simulink model "sysgen_oversample2x_2samples_per_clock"  (R2016b)
settings: Solver=VariableStepAuto  StartTime=0.0  StopTime=samples_per_channel*number_channels  RelTol=1e-3
PreLoadFcn:
  | setup
values from neighbouring files (symbols this model uses):
  filts = reshape(filt,number_subband,taps_per_chan)    [setup.m]
undefined symbols (not defined in the file or in its folder): j
libraries: xbsIndex_r4 x186, dspsigops x4, dspxfrm3 x4, hdlsllib x2
(part 1 of 3)
settings Model: Creator=mdewart  LastModifiedBy=mdewart

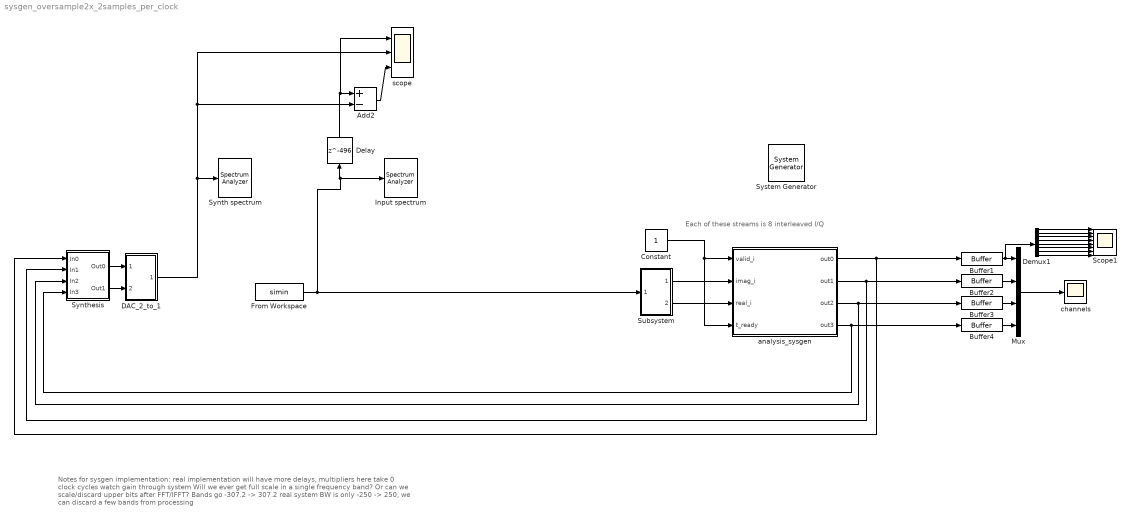
== system sysgen_oversample2x_2samples_per_clock ==
  note: Notes for sysgen implementation:
      |
      | real implementation will have more delays, multipliers here take 0 clock cycles
      |
      | watch gain through system
      |      Will we ever get full scale in a single frequency band?  Or can we scale/discard upper bits after FFT/IFFT?
      |
      | Bands go -307.2 -> 307.2  real system BW is only -250 -> 250, we can discard a few bands from processing
  note: Each of these streams is 8 interleaved I/Q
  " System Generator" : xbsIndex_r4/ System Generator  Tag=genX  xilinxfamily=kintexu  part=xcku040  speed=-2-e  package=ffva1156  synthesis_tool=Vivado  clock_wrapper=Clock Enables  directory=./netlist  proj_type=Vivado  Synth_file=Vivado Synthesis Defaults  Impl_file=Vivado Implementation Defaults  testbench=off  simulink_period=2  sysclk_period=10  dcm_input_clock_period=10  incr_netlist=off  trim_vbits=Everywhere in SubSystem  dbl_ovrd=According to Block Masks  core_generation=According to Block Masks  run_coregen=off  deprecated_control=off  eval_field=0  block_type=sysgen
  Add2 : Sum  Inputs=+-
  Buffer{1..4} (4 alike) : Buffer  N=8  TreatMby1Signals=One channel  OutputFrames=off
  Constant : Constant  SampleTime=2
  DAC_2_to_1 : Subsystem
  Delay : Delay  DelayLength=496  InitialCondition=0
  Demux1 : Demux  Outputs=8
  From Workspace : FromWorkspace  VariableName=simin  SampleTime=1  Interpolate=off  OutputAfterFinalValue=Cyclic repetition
  Input spectrum : SpectrumAnalyzer
  Mux : Mux
  Scope1 : Scope  NumInputPorts=8
  Subsystem : Subsystem
  Synth spectrum : SpectrumAnalyzer
  Synthesis : Subsystem
  analysis_sysgen : Subsystem
  channels : Scope
  scope : Scope  NumInputPorts=3
  wires:
  Mux/1 -> channels/1
  Buffer2/1 -> Mux/2
  Buffer3/1 -> Mux/3
  Buffer4/1 -> Mux/4
  Add2/1 -> scope/3
  DAC_2_to_1/1(Out1) -> Add2/2, scope/2, Synth spectrum/1
  Delay/1 -> Add2/1, scope/1
  Subsystem/1(imag) -> analysis_sysgen/2(imag_i)
  Subsystem/2(real) -> analysis_sysgen/3(real_i)
  Constant/1 -> analysis_sysgen/4(t_ready), analysis_sysgen/1(valid_i)
  Buffer1/1 -> Demux1/1, Mux/1
  From Workspace/1 -> Delay/1, Input spectrum/1, Subsystem/1(In1)
  Demux1/1 -> Scope1/1
  Demux1/2 -> Scope1/2
  Demux1/3 -> Scope1/3
  Demux1/4 -> Scope1/4
  Demux1/5 -> Scope1/5
  Demux1/6 -> Scope1/6
  Demux1/7 -> Scope1/7
  Demux1/8 -> Scope1/8
  analysis_sysgen/3(out2) -> Buffer3/1, Synthesis/3(In2)
  analysis_sysgen/4(out3) -> Synthesis/4(In3), Buffer4/1
  analysis_sysgen/2(out1) -> Buffer2/1, Synthesis/2(In1)
  analysis_sysgen/1(out0) -> Buffer1/1, Synthesis/1(In0)
  Synthesis/1(Out0) -> DAC_2_to_1/1(In1)
  Synthesis/2(Out1) -> DAC_2_to_1/2(In2)

== system sysgen_oversample2x_2samples_per_clock/DAC_2_to_1 ==
  In1 : Inport
  In2 : Inport  Port=2
  Add2 : Sum
  Delay7 : Delay  DelayLength=1  InitialCondition=0
  Upsample1 : dspsigops/Upsample  N=2  phase=0  RateOptions=Allow multirate processing  ic=0  mode=Unused parameter value
  Upsample2 : dspsigops/Upsample  N=2  phase=0  RateOptions=Allow multirate processing  ic=0  mode=Unused parameter value
  Out1 : Outport
  wires:
  In2/1 -> Upsample2/1
  Delay7/1 -> Add2/2
  In1/1 -> Upsample1/1
  Upsample1/1 -> Add2/1
  Add2/1 -> Out1/1
  Upsample2/1 -> Delay7/1

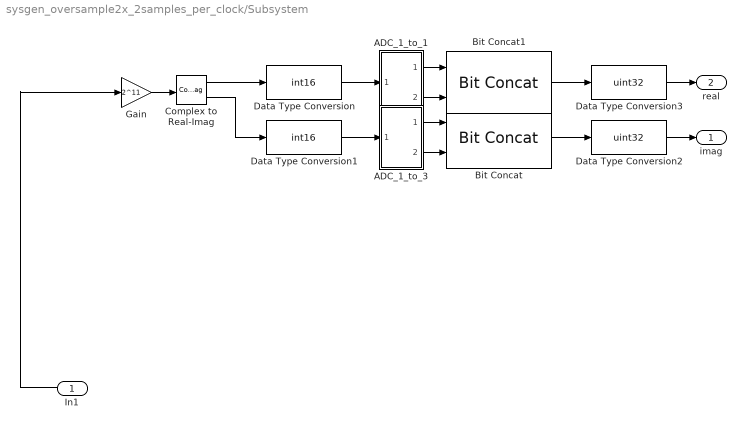
== system sysgen_oversample2x_2samples_per_clock/Subsystem ==
  In1 : Inport
  ADC_1_to_1 : Subsystem
  ADC_1_to_3 : Subsystem
  Bit Concat : hdlsllib/HDL Operations/Bit Concat  numInputs=2
  Bit Concat1 : hdlsllib/HDL Operations/Bit Concat  numInputs=2
  Complex to Real-Imag : ComplexToRealImag
  Data Type Conversion : DataTypeConversion  OutDataTypeStr=int16
  Data Type Conversion1 : DataTypeConversion  OutDataTypeStr=int16
  Data Type Conversion2 : DataTypeConversion  OutDataTypeStr=uint32  ConvertRealWorld=Stored Integer (SI)
  Data Type Conversion3 : DataTypeConversion  OutDataTypeStr=uint32  ConvertRealWorld=Stored Integer (SI)
  Gain : Gain  Gain=2^11
  imag : Outport
  real : Outport  Port=2
  wires:
  In1/1 -> Gain/1
  Data Type Conversion/1 -> ADC_1_to_1/1(In1)
  Complex to Real-Imag/1 -> Data Type Conversion/1
  ADC_1_to_3/2(Out2) -> Bit Concat/2
  Data Type Conversion1/1 -> ADC_1_to_3/1(In1)
  ADC_1_to_1/1(Out1) -> Bit Concat1/1
  Bit Concat/1 -> Data Type Conversion2/1
  ADC_1_to_3/1(Out1) -> Bit Concat/1
  ADC_1_to_1/2(Out2) -> Bit Concat1/2
  Complex to Real-Imag/2 -> Data Type Conversion1/1
  Gain/1 -> Complex to Real-Imag/1
  Bit Concat1/1 -> Data Type Conversion3/1
  Data Type Conversion2/1 -> imag/1
  Data Type Conversion3/1 -> real/1

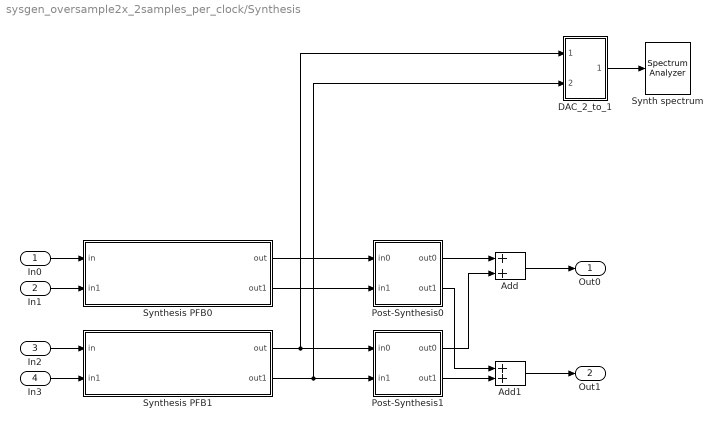
== system sysgen_oversample2x_2samples_per_clock/Synthesis ==
  In0 : Inport
  In1 : Inport  Port=2
  In2 : Inport  Port=3
  In3 : Inport  Port=4
  Add : Sum
  Add1 : Sum
  DAC_2_to_1 : Subsystem
  Post-Synthesis0 : Subsystem
  Post-Synthesis1 : Subsystem
  Synth spectrum : SpectrumAnalyzer
  Synthesis PFB0 : Subsystem
  Synthesis PFB1 : Subsystem
  Out0 : Outport
  Out1 : Outport  Port=2
  wires:
  Synthesis PFB0/2(out1) -> Post-Synthesis0/2(in1)
  Synthesis PFB0/1(out) -> Post-Synthesis0/1(in0)
  Post-Synthesis1/1(out0) -> Add/2
  Post-Synthesis0/2(out1) -> Add1/1
  Synthesis PFB1/2(out1) -> DAC_2_to_1/2(In2), Post-Synthesis1/2(in1)
  Post-Synthesis1/2(out1) -> Add1/2
  Synthesis PFB1/1(out) -> DAC_2_to_1/1(In1), Post-Synthesis1/1(in0)
  In2/1 -> Synthesis PFB1/1(in)
  In3/1 -> Synthesis PFB1/2(in1)
  In0/1 -> Synthesis PFB0/1(in)
  In1/1 -> Synthesis PFB0/2(in1)
  Post-Synthesis0/1(out0) -> Add/1
  Add1/1 -> Out1/1
  Add/1 -> Out0/1
  DAC_2_to_1/1(Out1) -> Synth spectrum/1

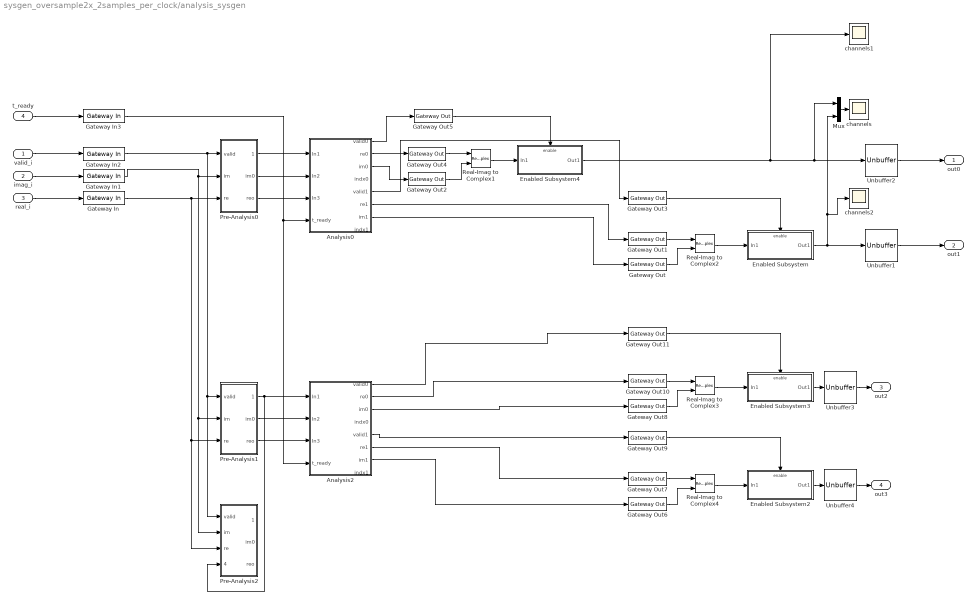
== system sysgen_oversample2x_2samples_per_clock/analysis_sysgen ==
  valid_i : Inport
  imag_i : Inport  Port=2
  real_i : Inport  Port=3
  t_ready : Inport  Port=4
  Analysis0 : Subsystem
  Analysis2 : Subsystem
  Enabled Subsystem : Subsystem  TreatAsAtomicUnit=on
  Enabled Subsystem2 : Subsystem  TreatAsAtomicUnit=on
  Enabled Subsystem3 : Subsystem  TreatAsAtomicUnit=on
  Enabled Subsystem4 : Subsystem  TreatAsAtomicUnit=on
  Gateway In : xbsIndex_r4/Gateway In  gui_display_data_type=Fixed-point  arith_type=Unsigned  n_bits=32  bin_pt=0  preci_type=Single  exp_width=8  frac_width=24  rows=1  columns=1  quantization="Round  (unbiased: +/- Inf)"  overflow=Saturate  period=2  UseAsADC=off  ADCChannel='1'  interface=None  automatic_assignment=on  address_offset=hex2dec('00')  intf_name=''  intf_description=''  default_value=0  timing_constraint=None  locs_specified=off  LOCs={}  io_standard={}  inherit_from_input=off  hdl_port=on  dbl_ovrd=off  block_type=gatewayin
  Gateway In1 : xbsIndex_r4/Gateway In  gui_display_data_type=Fixed-point  arith_type=Unsigned  n_bits=32  bin_pt=0  preci_type=Single  exp_width=8  frac_width=24  rows=1  columns=1  quantization="Round  (unbiased: +/- Inf)"  overflow=Saturate  period=2  UseAsADC=off  ADCChannel='1'  interface=None  automatic_assignment=on  address_offset=hex2dec('00')  intf_name=''  intf_description=''  default_value=0  timing_constraint=None  locs_specified=off  LOCs={}  io_standard={}  inherit_from_input=off  hdl_port=on  dbl_ovrd=off  block_type=gatewayin
  Gateway In2 : xbsIndex_r4/Gateway In  gui_display_data_type=Boolean  arith_type=Boolean  n_bits=1  bin_pt=0  preci_type=Single  exp_width=8  frac_width=24  rows=1  columns=1  quantization="Round  (unbiased: +/- Inf)"  overflow=Saturate  period=2  UseAsADC=off  ADCChannel='1'  interface=None  automatic_assignment=on  address_offset=hex2dec('00')  intf_name=''  intf_description=''  default_value=0  timing_constraint=None  locs_specified=off  LOCs={}  io_standard={}  inherit_from_input=off  hdl_port=on  dbl_ovrd=off  block_type=gatewayin
  Gateway In3 : xbsIndex_r4/Gateway In  gui_display_data_type=Boolean  arith_type=Boolean  n_bits=1  bin_pt=0  preci_type=Single  exp_width=8  frac_width=24  rows=1  columns=1  quantization="Round  (unbiased: +/- Inf)"  overflow=Saturate  period=2  UseAsADC=off  ADCChannel='1'  interface=None  automatic_assignment=on  address_offset=hex2dec('00')  intf_name=''  intf_description=''  default_value=0  timing_constraint=None  locs_specified=off  LOCs={}  io_standard={}  inherit_from_input=off  hdl_port=on  dbl_ovrd=off  block_type=gatewayin
  Gateway Out{,1..11} (12 alike) : xbsIndex_r4/Gateway Out  inherit_from_input=off  hdl_port=off  rows=1  columns=1  UseAsDAC=off  DACChannel='1'  interface=None  automatic_assignment=on  address_offset=hex2dec('00')  intf_name=''  intf_description=''  timing_constraint=None  locs_specified=off  LOCs={}  io_standard={}  block_type=gatewayout
  Mux : Mux  Inputs=2
  Pre-Analysis0 : Subsystem
  Pre-Analysis1 : Subsystem
  Pre-Analysis2 : Subsystem
  Real-Imag to Complex{1..4} (4 alike) : RealImagToComplex
  Unbuffer{1..4} (4 alike) : Unbuffer  SampleBasedProcessing=Same as frame based
  channels : Scope
  channels1 : Scope
  channels2 : Scope
  out0 : Outport
  out1 : Outport  Port=2
  out2 : Outport  Port=3
  out3 : Outport  Port=4
  wires:
  valid_i/1 -> Gateway In2/1
  t_ready/1 -> Gateway In3/1
  real_i/1 -> Gateway In/1
  imag_i/1 -> Gateway In1/1
  Enabled Subsystem/1(Out1) -> channels2/1, Mux/2, Unbuffer1/1
  Gateway Out1/1 -> Real-Imag to Complex2/1
  Gateway Out/1 -> Real-Imag to Complex2/2
  Real-Imag to Complex2/1 -> Enabled Subsystem/1(In1)
  Gateway Out3/1 -> Enabled Subsystem/Enable
  Gateway Out4/1 -> Real-Imag to Complex1/1
  Gateway Out2/1 -> Real-Imag to Complex1/2
  Analysis0/5(valid1) -> Gateway Out3/1
  Analysis0/6(re1) -> Gateway Out1/1
  Analysis0/7(im1) -> Gateway Out/1
  Gateway Out7/1 -> Real-Imag to Complex4/1
  Gateway Out6/1 -> Real-Imag to Complex4/2
  Real-Imag to Complex4/1 -> Enabled Subsystem2/1(In1)
  Gateway Out9/1 -> Enabled Subsystem2/Enable
  Gateway Out10/1 -> Real-Imag to Complex3/1
  Gateway Out8/1 -> Real-Imag to Complex3/2
  Gateway Out11/1 -> Enabled Subsystem3/Enable
  Real-Imag to Complex3/1 -> Enabled Subsystem3/1(In1)
  Analysis2/1(valid0) -> Gateway Out11/1
  Analysis2/2(re0) -> Gateway Out10/1
  Analysis2/5(valid1) -> Gateway Out9/1
  Gateway In2/1 -> Pre-Analysis1/1(valid), Pre-Analysis2/1(valid), Pre-Analysis0/1(valid)
  Gateway In1/1 -> Pre-Analysis1/2(im), Pre-Analysis2/2(im), Pre-Analysis0/2(im)
  Gateway In/1 -> Pre-Analysis2/3(re), Pre-Analysis1/3(re), Pre-Analysis0/3(re)
  Pre-Analysis0/3(reo) -> Analysis0/3(In3)
  Pre-Analysis0/2(im0) -> Analysis0/2(In2)
  Pre-Analysis0/1(valid0) -> Analysis0/1(In1)
  Gateway In3/1 -> Analysis2/4(t_ready), Analysis0/4(t_ready)
  Pre-Analysis1/3(reo) -> Analysis2/3(In3)
  Pre-Analysis1/2(im0) -> Analysis2/2(In2)
  Pre-Analysis1/1(valid0) -> Analysis2/1(In1), Pre-Analysis2/4(valid1)
  Real-Imag to Complex1/1 -> Enabled Subsystem4/1(In1)
  Gateway Out5/1 -> Enabled Subsystem4/Enable
  Unbuffer2/1 -> out0/1
  Unbuffer1/1 -> out1/1
  Enabled Subsystem3/1(Out1) -> Unbuffer3/1
  Unbuffer3/1 -> out2/1
  Enabled Subsystem2/1(Out1) -> Unbuffer4/1
  Unbuffer4/1 -> out3/1
  Analysis0/3(im0) -> Gateway Out2/1
  Analysis0/2(re0) -> Gateway Out4/1
  Analysis0/1(valid0) -> Gateway Out5/1
  Mux/1 -> channels/1
  Enabled Subsystem4/1(Out1) -> channels1/1, Mux/1, Unbuffer2/1
  Analysis2/3(im0) -> Gateway Out8/1
  Analysis2/6(re1) -> Gateway Out7/1
  Analysis2/7(im1) -> Gateway Out6/1

== system sysgen_oversample2x_2samples_per_clock/Subsystem/ADC_1_to_1 ==
  In1 : Inport
  Delay1 : Delay  DelayLength=1  InitialCondition=0
  Downsample : DownSample  RateOptions=Allow multirate processing
  Downsample1 : DownSample  RateOptions=Allow multirate processing
  Out1 : Outport
  Out2 : Outport  Port=2
  wires:
  Downsample/1 -> Out2/1
  In1/1 -> Downsample/1, Delay1/1
  Downsample1/1 -> Out1/1
  Delay1/1 -> Downsample1/1

== system sysgen_oversample2x_2samples_per_clock/Subsystem/ADC_1_to_3 ==
  In1 : Inport
  Delay1 : Delay  DelayLength=1  InitialCondition=0
  Downsample : DownSample  RateOptions=Allow multirate processing
  Downsample1 : DownSample  RateOptions=Allow multirate processing
  Out1 : Outport
  Out2 : Outport  Port=2
  wires:
  Delay1/1 -> Downsample1/1
  Downsample1/1 -> Out1/1
  In1/1 -> Delay1/1, Downsample/1
  Downsample/1 -> Out2/1

== system sysgen_oversample2x_2samples_per_clock/Synthesis/DAC_2_to_1 ==
  In1 : Inport
  In2 : Inport  Port=2
  Add2 : Sum
  Delay7 : Delay  DelayLength=1  InitialCondition=0
  Upsample1 : dspsigops/Upsample  N=2  phase=0  RateOptions=Allow multirate processing  ic=0  mode=Unused parameter value
  Upsample2 : dspsigops/Upsample  N=2  phase=0  RateOptions=Allow multirate processing  ic=0  mode=Unused parameter value
  Out1 : Outport
  wires:
  In2/1 -> Upsample2/1
  Delay7/1 -> Add2/2
  In1/1 -> Upsample1/1
  Upsample1/1 -> Add2/1
  Add2/1 -> Out1/1
  Upsample2/1 -> Delay7/1

== system sysgen_oversample2x_2samples_per_clock/Synthesis/Post-Synthesis0 ==
  note: Post-synthesis0 match timing to post-synthesis
  in0 : Inport
  in1 : Inport  Port=2
  out0 : Outport
  out1 : Outport  Port=2
  wires:
  in1/1 -> out1/1
  in0/1 -> out0/1

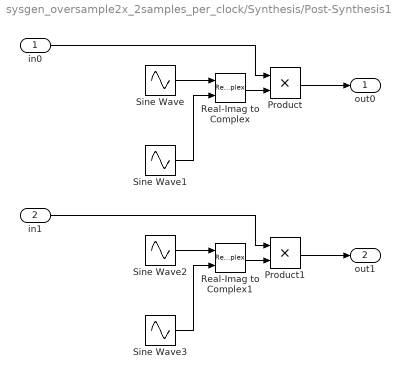
== system sysgen_oversample2x_2samples_per_clock/Synthesis/Post-Synthesis1 ==
  in0 : Inport
  in1 : Inport  Port=2
  Product : Product
  Product1 : Product
  Real-Imag to Complex : RealImagToComplex
  Real-Imag to Complex1 : RealImagToComplex
  Sine Wave : Sin  Frequency=2*pi/32  Phase=-pi/2  SampleTime=2
  Sine Wave1 : Sin  Amplitude=-1  Frequency=2*pi/32  SampleTime=2
  Sine Wave2 : Sin  Frequency=2*pi/32  Phase=-pi/2+pi/16  SampleTime=2
  Sine Wave3 : Sin  Amplitude=-1  Frequency=2*pi/32  Phase=0+pi/16  SampleTime=2
  out0 : Outport
  out1 : Outport  Port=2
  wires:
  in0/1 -> Product/1
  ? -> ?
  ? -> ?
  Sine Wave/1 -> Real-Imag to Complex/1
  Sine Wave1/1 -> Real-Imag to Complex/2
  in1/1 -> Product1/1
  Sine Wave2/1 -> Real-Imag to Complex1/1
  Sine Wave3/1 -> Real-Imag to Complex1/2
  Real-Imag to Complex1/1 -> Product1/2
  Real-Imag to Complex/1 -> Product/2
  Product1/1 -> out1/1
  Product/1 -> out0/1

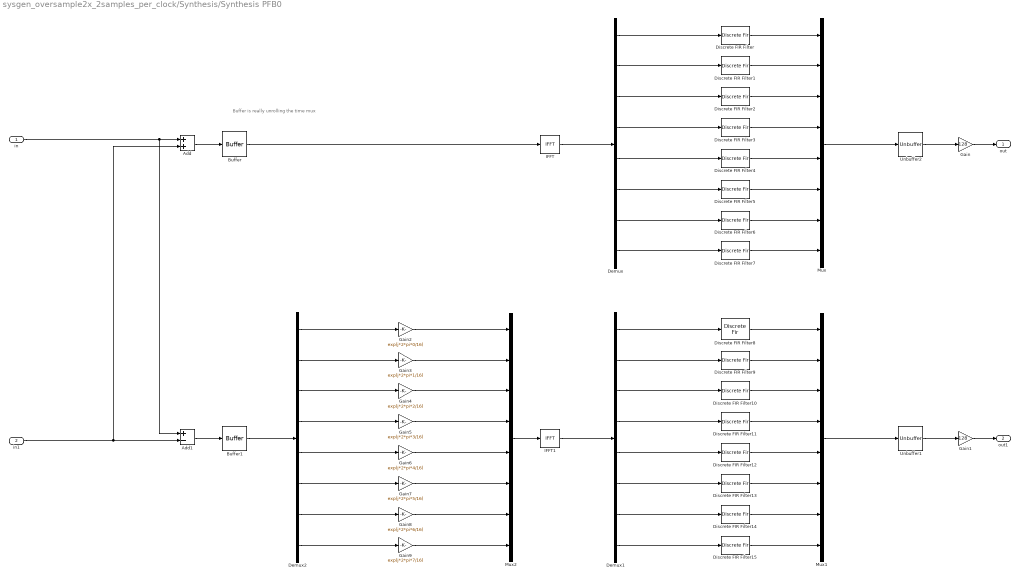
== system sysgen_oversample2x_2samples_per_clock/Synthesis/Synthesis PFB0 ==
  note: Buffer is really unrolling the time mux
  in : Inport
  in1 : Inport  Port=2
  Add : Sum
  Add1 : Sum  Inputs=+-
  Buffer : Buffer  N=8  TreatMby1Signals=One channel  OutputFrames=off
  Buffer1 : Buffer  N=8  TreatMby1Signals=One channel  OutputFrames=off
  Demux : Demux  Outputs=8
  Demux1 : Demux  Outputs=8
  Demux2 : Demux  Outputs=8
  Discrete FIR Filter : DiscreteFir  Coefficients=filts(1,:)
  Discrete FIR Filter1 : DiscreteFir  Coefficients=filts(3,:)
  Discrete FIR Filter10 : DiscreteFir  Coefficients=filts(6,:)
  Discrete FIR Filter11 : DiscreteFir  Coefficients=filts(8,:)
  Discrete FIR Filter12 : DiscreteFir  Coefficients=filts(10,:)
  Discrete FIR Filter13 : DiscreteFir  Coefficients=filts(12,:)
  Discrete FIR Filter14 : DiscreteFir  Coefficients=filts(14,:)
  Discrete FIR Filter15 : DiscreteFir  Coefficients=filts(16,:)
  Discrete FIR Filter2 : DiscreteFir  Coefficients=filts(5,:)
  Discrete FIR Filter3 : DiscreteFir  Coefficients=filts(7,:)
  Discrete FIR Filter4 : DiscreteFir  Coefficients=filts(9,:)
  Discrete FIR Filter5 : DiscreteFir  Coefficients=filts(11,:)
  Discrete FIR Filter6 : DiscreteFir  Coefficients=filts(13,:)
  Discrete FIR Filter7 : DiscreteFir  Coefficients=filts(15,:)
  Discrete FIR Filter8 : DiscreteFir  Coefficients=filts(2,:)
  Discrete FIR Filter9 : DiscreteFir  Coefficients=filts(4,:)
  Gain : Gain  Gain=128
  Gain1 : Gain  Gain=128
  Gain2 : Gain  Gain=exp(j*2*pi*0/16)
  Gain3 : Gain  Gain=exp(j*2*pi*1/16)
  Gain4 : Gain  Gain=exp(j*2*pi*2/16)
  Gain5 : Gain  Gain=exp(j*2*pi*3/16)
  Gain6 : Gain  Gain=exp(j*2*pi*4/16)
  Gain7 : Gain  Gain=exp(j*2*pi*5/16)
  Gain8 : Gain  Gain=exp(j*2*pi*6/16)
  Gain9 : Gain  Gain=exp(j*2*pi*7/16)
  IFFT : dspxfrm3/IFFT  FFTImplementation=Auto  CompMethod=Table lookup  TableOpt=NEW  TableOptActive=Speed  BitRevOrder=off  cs_in=off  Normalize=on  InheritFFTLength=on  FFTLength=64  WrapInput=on  mode=Complex  outSamplingMode=Sample based  roundingMode=Floor  overflowMode=off  firstCoeffDataTypeStr=Inherit: Same word length as input  firstCoeffLastDataTypeStr=Inherit: Same word length as input  outputMin=[]  outputMax=[]
  IFFT1 : dspxfrm3/IFFT  FFTImplementation=Auto  CompMethod=Table lookup  TableOpt=NEW  TableOptActive=Speed  BitRevOrder=off  cs_in=off  Normalize=on  InheritFFTLength=on  FFTLength=64  WrapInput=on  mode=Complex  outSamplingMode=Sample based  roundingMode=Floor  overflowMode=off  firstCoeffDataTypeStr=Inherit: Same word length as input  firstCoeffLastDataTypeStr=Inherit: Same word length as input  outputMin=[]  outputMax=[]
  Mux : Mux  Inputs=8
  Mux1 : Mux  Inputs=8
  Mux2 : Mux  Inputs=8
  Unbuffer1 : Unbuffer  SampleBasedProcessing=Same as frame based
  Unbuffer2 : Unbuffer  SampleBasedProcessing=Same as frame based
  out : Outport
  out1 : Outport  Port=2
  wires:
  Discrete FIR Filter7/1 -> Mux/8
  IFFT/1 -> Demux/1
  Demux/2 -> Discrete FIR Filter1/1
  Demux/7 -> Discrete FIR Filter6/1
  Demux/5 -> Discrete FIR Filter4/1
  Demux/8 -> Discrete FIR Filter7/1
  Demux/3 -> Discrete FIR Filter2/1
  Demux/1 -> Discrete FIR Filter/1
  Demux/6 -> Discrete FIR Filter5/1
  Discrete FIR Filter5/1 -> Mux/6
  Discrete FIR Filter/1 -> Mux/1
  Discrete FIR Filter4/1 -> Mux/5
  Discrete FIR Filter2/1 -> Mux/3
  Discrete FIR Filter1/1 -> Mux/2
  Discrete FIR Filter3/1 -> Mux/4
  Discrete FIR Filter6/1 -> Mux/7
  Demux/4 -> Discrete FIR Filter3/1
  Mux/1 -> Unbuffer2/1
  Unbuffer2/1 -> Gain/1
  Add/1 -> Buffer/1
  in/1 -> Add1/1, Add/1
  Discrete FIR Filter15/1 -> Mux1/8
  IFFT1/1 -> Demux1/1
  Demux1/2 -> Discrete FIR Filter9/1
  Demux1/7 -> Discrete FIR Filter14/1
  Demux1/5 -> Discrete FIR Filter12/1
  Demux1/8 -> Discrete FIR Filter15/1
  Demux1/3 -> Discrete FIR Filter10/1
  Demux1/1 -> Discrete FIR Filter8/1
  Demux1/6 -> Discrete FIR Filter13/1
  Discrete FIR Filter13/1 -> Mux1/6
  Discrete FIR Filter8/1 -> Mux1/1
  Discrete FIR Filter12/1 -> Mux1/5
  Discrete FIR Filter10/1 -> Mux1/3
  Discrete FIR Filter9/1 -> Mux1/2
  Discrete FIR Filter11/1 -> Mux1/4
  Discrete FIR Filter14/1 -> Mux1/7
  Demux1/4 -> Discrete FIR Filter11/1
  Mux1/1 -> Unbuffer1/1
  Unbuffer1/1 -> Gain1/1
  Add1/1 -> Buffer1/1
  in1/1 -> Add/2, Add1/2
  Mux2/1 -> IFFT1/1
  Demux2/4 -> Gain5/1
  Demux2/7 -> Gain8/1
  Demux2/8 -> Gain9/1
  Demux2/1 -> Gain2/1
  Demux2/5 -> Gain6/1
  Demux2/3 -> Gain4/1
  Demux2/6 -> Gain7/1
  Demux2/2 -> Gain3/1
  Gain2/1 -> Mux2/1
  Gain3/1 -> Mux2/2
  Gain4/1 -> Mux2/3
  Gain5/1 -> Mux2/4
  Gain6/1 -> Mux2/5
  Gain7/1 -> Mux2/6
  Gain8/1 -> Mux2/7
  Gain9/1 -> Mux2/8
  Gain/1 -> out/1
  Gain1/1 -> out1/1
  Buffer/1 -> IFFT/1
  Buffer1/1 -> Demux2/1

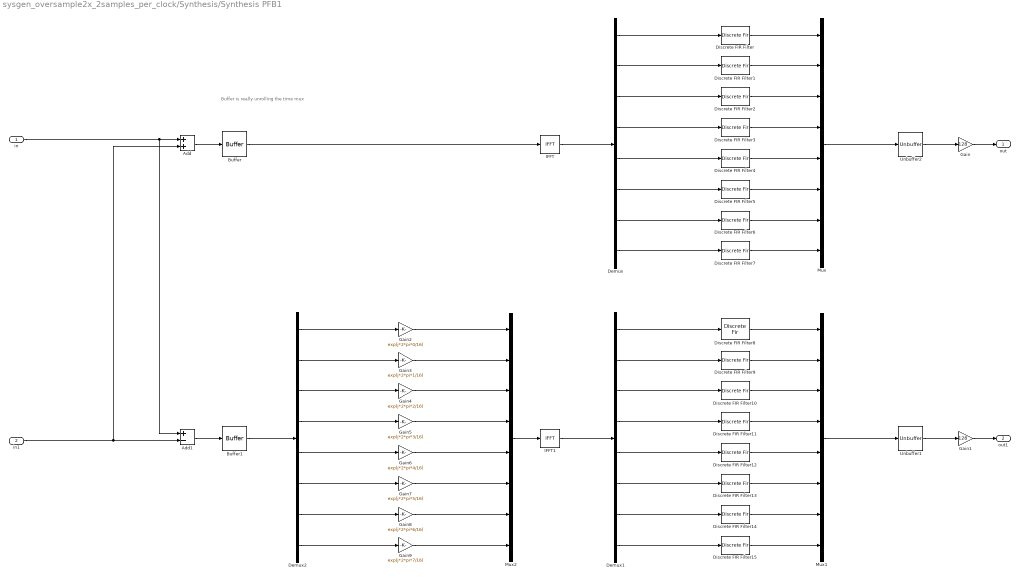
== system sysgen_oversample2x_2samples_per_clock/Synthesis/Synthesis PFB1 ==
  note: Buffer is really unrolling the time mux
  in : Inport
  in1 : Inport  Port=2
  Add : Sum
  Add1 : Sum  Inputs=+-
  Buffer : Buffer  N=8  TreatMby1Signals=One channel  OutputFrames=off
  Buffer1 : Buffer  N=8  TreatMby1Signals=One channel  OutputFrames=off
  Demux : Demux  Outputs=8
  Demux1 : Demux  Outputs=8
  Demux2 : Demux  Outputs=8
  Discrete FIR Filter : DiscreteFir  Coefficients=filts(1,:)
  Discrete FIR Filter1 : DiscreteFir  Coefficients=filts(3,:)
  Discrete FIR Filter10 : DiscreteFir  Coefficients=filts(6,:)
  Discrete FIR Filter11 : DiscreteFir  Coefficients=filts(8,:)
  Discrete FIR Filter12 : DiscreteFir  Coefficients=filts(10,:)
  Discrete FIR Filter13 : DiscreteFir  Coefficients=filts(12,:)
  Discrete FIR Filter14 : DiscreteFir  Coefficients=filts(14,:)
  Discrete FIR Filter15 : DiscreteFir  Coefficients=filts(16,:)
  Discrete FIR Filter2 : DiscreteFir  Coefficients=filts(5,:)
  Discrete FIR Filter3 : DiscreteFir  Coefficients=filts(7,:)
  Discrete FIR Filter4 : DiscreteFir  Coefficients=filts(9,:)
  Discrete FIR Filter5 : DiscreteFir  Coefficients=filts(11,:)
  Discrete FIR Filter6 : DiscreteFir  Coefficients=filts(13,:)
  Discrete FIR Filter7 : DiscreteFir  Coefficients=filts(15,:)
  Discrete FIR Filter8 : DiscreteFir  Coefficients=filts(2,:)
  Discrete FIR Filter9 : DiscreteFir  Coefficients=filts(4,:)
  Gain : Gain  Gain=128
  Gain1 : Gain  Gain=128
  Gain2 : Gain  Gain=exp(j*2*pi*0/16)
  Gain3 : Gain  Gain=exp(j*2*pi*1/16)
  Gain4 : Gain  Gain=exp(j*2*pi*2/16)
  Gain5 : Gain  Gain=exp(j*2*pi*3/16)
  Gain6 : Gain  Gain=exp(j*2*pi*4/16)
  Gain7 : Gain  Gain=exp(j*2*pi*5/16)
  Gain8 : Gain  Gain=exp(j*2*pi*6/16)
  Gain9 : Gain  Gain=exp(j*2*pi*7/16)
  IFFT : dspxfrm3/IFFT  FFTImplementation=Auto  CompMethod=Table lookup  TableOpt=NEW  TableOptActive=Speed  BitRevOrder=off  cs_in=off  Normalize=on  InheritFFTLength=on  FFTLength=64  WrapInput=on  mode=Complex  outSamplingMode=Sample based  roundingMode=Floor  overflowMode=off  firstCoeffDataTypeStr=Inherit: Same word length as input  firstCoeffLastDataTypeStr=Inherit: Same word length as input  outputMin=[]  outputMax=[]
  IFFT1 : dspxfrm3/IFFT  FFTImplementation=Auto  CompMethod=Table lookup  TableOpt=NEW  TableOptActive=Speed  BitRevOrder=off  cs_in=off  Normalize=on  InheritFFTLength=on  FFTLength=64  WrapInput=on  mode=Complex  outSamplingMode=Sample based  roundingMode=Floor  overflowMode=off  firstCoeffDataTypeStr=Inherit: Same word length as input  firstCoeffLastDataTypeStr=Inherit: Same word length as input  outputMin=[]  outputMax=[]
  Mux : Mux  Inputs=8
  Mux1 : Mux  Inputs=8
  Mux2 : Mux  Inputs=8
  Unbuffer1 : Unbuffer  SampleBasedProcessing=Same as frame based
  Unbuffer2 : Unbuffer  SampleBasedProcessing=Same as frame based
  out : Outport
  out1 : Outport  Port=2
  wires:
  Discrete FIR Filter7/1 -> Mux/8
  IFFT/1 -> Demux/1
  Demux/2 -> Discrete FIR Filter1/1
  Demux/7 -> Discrete FIR Filter6/1
  Demux/5 -> Discrete FIR Filter4/1
  Demux/8 -> Discrete FIR Filter7/1
  Demux/3 -> Discrete FIR Filter2/1
  Demux/1 -> Discrete FIR Filter/1
  Demux/6 -> Discrete FIR Filter5/1
  Discrete FIR Filter5/1 -> Mux/6
  Discrete FIR Filter/1 -> Mux/1
  Discrete FIR Filter4/1 -> Mux/5
  Discrete FIR Filter2/1 -> Mux/3
  Discrete FIR Filter1/1 -> Mux/2
  Discrete FIR Filter3/1 -> Mux/4
  Discrete FIR Filter6/1 -> Mux/7
  Demux/4 -> Discrete FIR Filter3/1
  Mux/1 -> Unbuffer2/1
  Unbuffer2/1 -> Gain/1
  Add/1 -> Buffer/1
  in/1 -> Add1/1, Add/1
  Discrete FIR Filter15/1 -> Mux1/8
  IFFT1/1 -> Demux1/1
  Demux1/2 -> Discrete FIR Filter9/1
  Demux1/7 -> Discrete FIR Filter14/1
  Demux1/5 -> Discrete FIR Filter12/1
  Demux1/8 -> Discrete FIR Filter15/1
  Demux1/3 -> Discrete FIR Filter10/1
  Demux1/1 -> Discrete FIR Filter8/1
  Demux1/6 -> Discrete FIR Filter13/1
  Discrete FIR Filter13/1 -> Mux1/6
  Discrete FIR Filter8/1 -> Mux1/1
  Discrete FIR Filter12/1 -> Mux1/5
  Discrete FIR Filter10/1 -> Mux1/3
  Discrete FIR Filter9/1 -> Mux1/2
  Discrete FIR Filter11/1 -> Mux1/4
  Discrete FIR Filter14/1 -> Mux1/7
  Demux1/4 -> Discrete FIR Filter11/1
  Mux1/1 -> Unbuffer1/1
  Unbuffer1/1 -> Gain1/1
  Add1/1 -> Buffer1/1
  in1/1 -> Add/2, Add1/2
  Mux2/1 -> IFFT1/1
  Demux2/4 -> Gain5/1
  Demux2/7 -> Gain8/1
  Demux2/8 -> Gain9/1
  Demux2/1 -> Gain2/1
  Demux2/5 -> Gain6/1
  Demux2/3 -> Gain4/1
  Demux2/6 -> Gain7/1
  Demux2/2 -> Gain3/1
  Gain2/1 -> Mux2/1
  Gain3/1 -> Mux2/2
  Gain4/1 -> Mux2/3
  Gain5/1 -> Mux2/4
  Gain6/1 -> Mux2/5
  Gain7/1 -> Mux2/6
  Gain8/1 -> Mux2/7
  Gain9/1 -> Mux2/8
  Gain/1 -> out/1
  Gain1/1 -> out1/1
  Buffer/1 -> IFFT/1
  Buffer1/1 -> Demux2/1
